simulink model "AutoFollow_Simulation"  (R2014a)
settings: Solver=ode45  StartTime=0.0  StopTime=50  FixedStep=0.05  MaxStep=0.06  RelTol=1e-3
model workspace (MAT data in the model file):
  Sig = Simulink.Signal
  Sig.DataType = 'auto'
  Sig.Dimensions = -1
  Sig.DimensionsMode = 'auto'
  Sig.Complexity = 'auto'
  Sig.SampleTime = -1
  Sig.SamplingMode = 'auto'
undefined symbols (not defined in the file or in its folder): IC, quadModel
libraries: simulink x4, commnoisgen2 x2
(part 1 of 2)
Description:
  | This is a configurable quadcopter simulation.
  | This Simulink model demonstates position control.
  | 
  | Additional quadcopter modeling and simulation materials available at:
  | github.com/dch33/Quad-Sim
  | 
  | Copyright (C) 2014 D. Hartman, K. Landis, S. Moreno, J. Kim, M. Mehrer
  | 
  | License:
  |     This program is free software: you can redistribute it and/or modify
  |     it under the terms of the GNU LESSER GENERAL PUBLIC LICENSE as published by
  |     the Free Software Foundation, either version 3 of the License, or
  |     (at your option) any later version.
  | 
  |     This program is distributed in the hope that it will be useful,
  |     but WITHOUT ANY WARRANTY; without even the implied warranty of
  |     MERCHANTABILITY or FITNESS FOR A PARTICULAR PURPOSE.  See the
  |     GNU General Public License for more details.
  | 
  |     You should have received a copy of the GNU LESSER GENERAL PUBLIC LICENSE
  |     along with this program.  If not, see <http://www.gnu.org/licenses/>.
settings Model: ModifiedComment=matthew -- Tue May 10 21:44:44 2016 -- Version 1.8  Creator=David Hartman  LastModifiedBy=jpacker
settings Model: ModifiedHistory=|
  | matthew -- Tue May 10 21:44:44 2016 -- Version 1.8
  | 
  | 
  | matthew -- Tue May 10 21:39:59 2016 -- Version 1.7
  | 
  | 
  | matthew -- Sun May 01 12:50:44 2016 -- Version 1.6
  | 
  | 
  | davidhartman -- Fri Jun 06 22:59:54 2014 -- Version 1.5
settings DataIOCC: LimitDataPoints=off  SignalLogging=off
settings OptimizationCC: InlineParams=on
settings DebuggingCC: MergeDetectMultiDrivingBlocksExec=error  UniqueDataStoreMsg=warning  StateNameClashWarn=warning  StrictBusMsg=ErrorOnBusTreatedAsVector

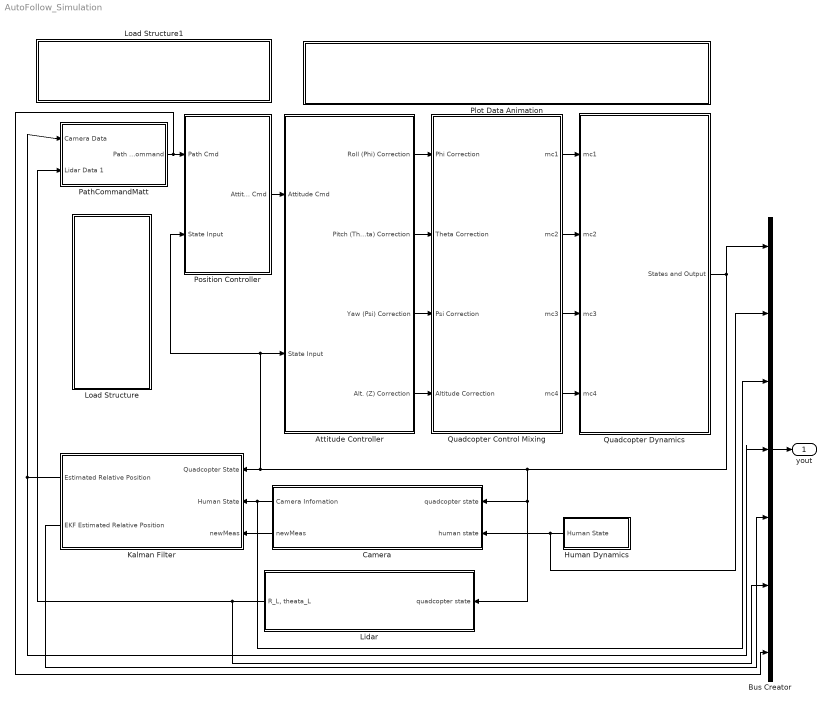
== system AutoFollow_Simulation ==
  Attitude Controller : Subsystem
  Bus Creator : BusCreator  Inputs=7
  Camera : Subsystem
  Human Dynamics : Subsystem
  Kalman Filter : Subsystem
  Lidar : Subsystem
  Load Structure : Subsystem
      settings: OpenFcn=|
      | uiopen('load')
      | if ((exist('IC')==1) && (exist('quadModel')==1) && (exist('path')==1))
      | set_param(bdroot, 'SimulationCommand', 'update')
      | end
      mask Display: fprintf('LOAD:\nTimeseries\nPath\nCommands,\nQuadcopter\nModel, Or\nInitial\nConditions');
  Load Structure1 : Subsystem
      settings: OpenFcn=|
      | if (exist('IC')==1 && exist('quadModel')==1 && exist('yout') && exist('tout'))
      | saveSimResults()
      | else
      | msgbox('No Data To Save!')
      | end
      mask Display: fprintf('SAVE:\nSimulation\nResults');
  "PathCommandMatt " : Subsystem
  Plot Data Animation : Subsystem
      settings: OpenFcn=|
      | if exist('QuadAnim4') == 2,
      |     if exist('yout')
      | 	run('QuadAnim4');
      |     else
      |     msgbox('Simulation must be run before data can be plotted.');
      |     end
      | else                                                                          msgbox('The desired GUI must be first added to MATLABs path.')
      | end
      mask Display: fprintf('OPEN GUI: Flight Animation')
  Position Controller : Subsystem
  Quadcopter Control Mixing : Subsystem
      mask Display:
      | modelLoaded = evalin('base','exist(''quadModel'',''var'')');
      | if (modelLoaded==1)
      |     if (evalin('base','quadModel.plusConfig'))
      |     fprintf([' \n' ' \n'  'Configuration "+"']);
      |     else if (~evalin('base','quadModel.plusConfig'))
      |         fprintf([' \n' ' \n' 'Configuration "X"']);
      |         end
      |     end
      | else
      |     fprintf([' \n' ' \n'  'Model Not Loaded']);
      | end
  Quadcopter Dynamics : Subsystem
  yout : Outport
  wires:
  Quadcopter Control Mixing/1(mc1) -> Quadcopter Dynamics/1(mc1)
  Quadcopter Control Mixing/2(mc2) -> Quadcopter Dynamics/2(mc2)
  Quadcopter Control Mixing/3(mc3) -> Quadcopter Dynamics/3(mc3)
  Quadcopter Control Mixing/4(mc4) -> Quadcopter Dynamics/4(mc4)
  Quadcopter Dynamics/1(States and Output) -> Lidar/1(quadcopter state), Camera/1(quadcopter state), Kalman Filter/1(Quadcopter State), Attitude Controller/2(State Input), Position Controller/2(State Input), Bus Creator/1
  Attitude Controller/1(Roll (Phi) Correction) -> Quadcopter Control Mixing/1(Phi Correction)
  Attitude Controller/2(Pitch (Theta) Correction) -> Quadcopter Control Mixing/2(Theta Correction)
  Attitude Controller/3(Yaw (Psi) Correction) -> Quadcopter Control Mixing/3(Psi Correction)
  Attitude Controller/4(Alt. (Z) Correction) -> Quadcopter Control Mixing/4(Altitude Correction)
  Position Controller/1(Attitude Cmd) -> Attitude Controller/1(Attitude Cmd)
  "PathCommandMatt "/1("Path Command ") -> Bus Creator/7, Position Controller/1(Path Cmd)
  Human Dynamics/1(Human State) -> Bus Creator/2, Camera/2(human state)
  Camera/1(Camera Infomation) -> Bus Creator/3, Kalman Filter/2(Human State)
  Bus Creator/1 -> yout/1
  Lidar/1("R_L, theata_L") -> "PathCommandMatt "/2(Lidar Data 1), Bus Creator/6
  Kalman Filter/1(Estimated Relative Position) -> "PathCommandMatt "/1("Camera Data "), Bus Creator/4
  Kalman Filter/2(EKF Estimated Relative Position) -> Bus Creator/5
  Camera/2(newMeas) -> Kalman Filter/3(newMeas)

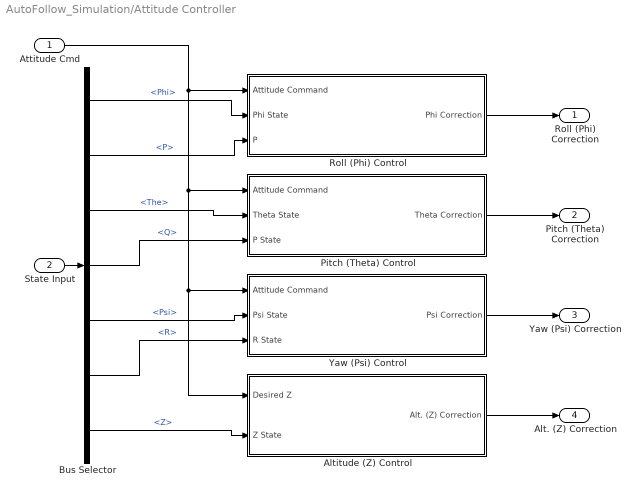
== system AutoFollow_Simulation/Attitude Controller ==
  Attitude Cmd : Inport
  State Input : Inport  Port=2
  Altitude (Z) Control : Subsystem  mask{Kpz=2, Kiz=1.1, Kdz=3.3, LimitOutput=on, USat=1, LSat=-1, GOffset=(sqrt((quadModel.mass*quadModel.g)/(4*quadModel.ct))-quadModel.b)/quadModel.cr}
      mask prompts: Kpz "Kp"; Kiz "Ki"; Kdz "Kd"; LimitOutput "Integral Saturation?"; USat "Upper saturation limit:"; LSat "Lower saturation limit:"; GOffset "Gravity Feedforward"
      mask help:
      | Adjust PID controller gains through this mask interface, or "look under mask" for more detailed adjustments.
      |
      | Note: Gravity Offset will not appear on block face as a value until simulation is run if it is the result of a formula involving the quadcopter model parameters.
      mask TypeOptions Kpz: Kpz/Gain
      mask TypeOptions Kiz: Kiz/Gain
      mask TypeOptions Kdz: Kdz/Gain
      mask TypeOptions LimitOutput:
      | Integrator
      | Limited/LimitOutput
      mask TypeOptions USat:
      | Integrator
      | Limited/UpperSaturationLimit
      mask TypeOptions LSat:
      | Integrator
      | Limited/LowerSaturationLimit
      mask TypeOptions GOffset: Gravity Offset (Level Flight)/Value
      mask Display:
      | fprintf(['Gravity Offset = ' num2str(GOffset) '\n' ...
      |     'Kp = ' num2str(Kpz) '\n' ...
      |     'Ki = ' num2str(Kiz) '\n' ...
      |     'Kd = ' num2str(Kdz) '\n' ...
      |     'Integral Saturation: ' LimitOutput]);
      | if strcmp(LimitOutput,'on')
      |     fprintf([' \n' ' \n' ' \n' ' \n' ' \n' '\n' ...
      |         'Limits: ' num2str(USat) ' to ' num2str(LSat)]);
      | end
  Bus Selector : BusSelector  OutputSignals=Phi,P,The,Q,Psi,R,Z
  Pitch (Theta) Control : Subsystem  mask{Kpt=2, Kit=1.1, Kdt=1.2, LimitOutput=on, USat=1, LSat=-1}
      mask prompts: Kpt "Kp"; Kit "Ki"; Kdt "Kd"; LimitOutput "Integral Saturation?"; USat "Upper saturation limit:"; LSat "Lower saturation limit:"
      mask help: Adjust PID controller gains through this mask interface, or "look under mask" for more detailed adjustments.
      mask TypeOptions Kpt: Kpt/Gain
      mask TypeOptions Kit: Kit/Gain
      mask TypeOptions Kdt: Kdt/Gain
      mask TypeOptions LimitOutput:
      | Integrator
      | Limited/LimitOutput
      mask TypeOptions USat:
      | Integrator
      | Limited/UpperSaturationLimit
      mask TypeOptions LSat:
      | Integrator
      | Limited/LowerSaturationLimit
      mask Display:
      | fprintf(['Kp = ' num2str(Kpt) '\n' ...
      |     'Ki = ' num2str(Kit) '\n' ...
      |     'Kd = ' num2str(Kdt) '\n' ...
      |     'Integral Saturation: ' LimitOutput]);
      | if strcmp(LimitOutput,'on')
      |     fprintf([' \n' ' \n' ' \n' ' \n' '\n' ...
      |         'Limits: ' num2str(USat) ' to ' num2str(LSat)]);
      | end
  "Roll (Phi) Control " : Subsystem  mask{Kpp=2.0, Kip=1.1, Kdp=1.2, LimitOutput=on, USat=1, LSat=-1}
      mask prompts: Kpp "Kp"; Kip "Ki"; Kdp "Kd"; LimitOutput "Integral Saturation:"; USat "Upper saturation limit:"; LSat "Lower saturation limit:"
      mask help:
      | Adjust PID controller gains through this mask interface, or "look under mask"
      | for more detailed adjustments.
      mask TypeOptions Kpp: Kpp/Gain
      mask TypeOptions Kip: Kip/Gain
      mask TypeOptions Kdp: Kdp/Gain
      mask TypeOptions LimitOutput:
      | Integrator
      | Limited/LimitOutput
      mask TypeOptions USat:
      | Integrator
      | Limited/UpperSaturationLimit
      mask TypeOptions LSat:
      | Integrator
      | Limited/LowerSaturationLimit
      mask Display:
      | fprintf(['Kp = ' num2str(Kpp) '\n' ...
      |     'Ki = ' num2str(Kip) '\n' ...
      |     'Kd = ' num2str(Kdp) '\n'...
      |     'Integral Saturation: ' LimitOutput]);
      | if strcmp(LimitOutput,'on')
      |     fprintf([' \n' ' \n' ' \n' ' \n' '\n' ...
      |         'Limits: ' num2str(USat) ' to ' num2str(LSat)]);
      | end
  Yaw (Psi) Control : Subsystem  mask{Kps=4, Kis=0.5, Kds=3.5, LimitOutput=on, USat=1, LSat=-1}
      mask prompts: Kps "Kp"; Kis "Ki"; Kds "Kd"; LimitOutput "Integral Saturation?"; USat "Upper saturation limit:"; LSat "Lower saturation limit:"
      mask help: Adjust PID controller gains through this mask interface, or "look under mask" for more detailed adjustments.
      mask TypeOptions Kps: Kps/Gain
      mask TypeOptions Kis: Kit/Gain
      mask TypeOptions Kds: Kds/Gain
      mask TypeOptions LimitOutput:
      | Integrator
      | Limited/LimitOutput
      mask TypeOptions USat:
      | Integrator
      | Limited/UpperSaturationLimit
      mask TypeOptions LSat:
      | Integrator
      | Limited/LowerSaturationLimit
      mask Display:
      | fprintf(['Kp = ' num2str(Kps) '\n' ...
      |     'Ki = ' num2str(Kis) '\n' ...
      |     'Kd = ' num2str(Kds) '\n' ...
      |     'Integral Saturation: ' LimitOutput]);
      | if strcmp(LimitOutput,'on')
      |     fprintf([' \n' ' \n' ' \n' ' \n' '\n' ...
      |         'Limits: ' num2str(USat) ' to ' num2str(LSat)]);
      | end
  Roll (Phi) Correction : Outport
  Pitch (Theta) Correction : Outport  Port=2
  Yaw (Psi) Correction : Outport  Port=3
  Alt. (Z) Correction : Outport  Port=4
  wires:
  "Roll (Phi) Control "/1(Phi Correction) -> Roll (Phi) Correction/1
  Bus Selector/1 -> "Roll (Phi) Control "/2(Phi State)  "<Phi>"
  State Input/1 -> Bus Selector/1
  Pitch (Theta) Control/1(Theta Correction) -> Pitch (Theta) Correction/1
  Yaw (Psi) Control/1(Psi Correction) -> Yaw (Psi) Correction/1
  Bus Selector/5 -> Yaw (Psi) Control/2(Psi State)  "<Psi>"
  Altitude (Z) Control/1(Alt. (Z) Correction) -> Alt. (Z) Correction/1
  Bus Selector/7 -> Altitude (Z) Control/2(Z State)  "<Z>"
  Attitude Cmd/1 -> Altitude (Z) Control/1(Desired Z), Yaw (Psi) Control/1(Attitude Command), Pitch (Theta) Control/1(Attitude Command), "Roll (Phi) Control "/1("Attitude Command ")
  Bus Selector/3 -> Pitch (Theta) Control/2(Theta State)  "<The>"
  Bus Selector/2 -> "Roll (Phi) Control "/3(P)  "<P>"
  Bus Selector/4 -> Pitch (Theta) Control/3(P State)  "<Q>"
  Bus Selector/6 -> Yaw (Psi) Control/3(R State)  "<R>"

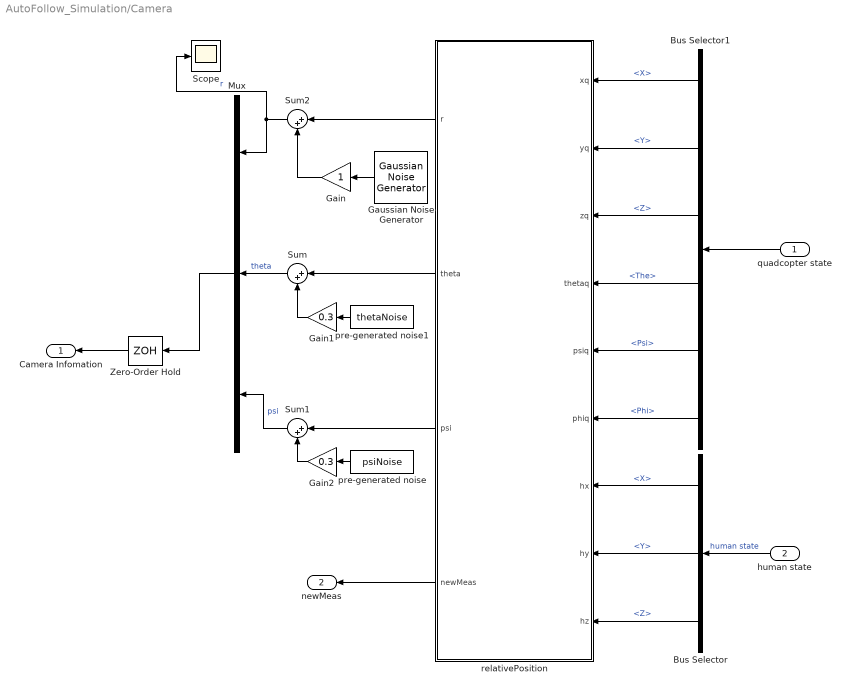
== system AutoFollow_Simulation/Camera ==
  quadcopter state : Inport
  human state : Inport  Port=2
  Bus Selector : BusSelector  OutputSignals=X,Y,Z
  Bus Selector1 : BusSelector  OutputSignals=X,Y,Z,The,Psi,Phi
  Gain : Gain
  Gain1 : Gain  Gain=0.3
  Gain2 : Gain  Gain=0.3
  Gaussian Noise Generator : commnoisgen2/Gaussian Noise Generator  m=0  d=1  s=35  Ts=1  frameBased=off  sampPerFrame=1  orient=off  outDataType=double
  Mux : Mux  Inputs=3
  Scope : Scope
  Sum : Sum  Inputs=|++
  Sum1 : Sum  Inputs=|++
  Sum2 : Sum  Inputs=|++
  Zero-Order Hold : ZeroOrderHold  SampleTime=0.05
  pre-generated noise : FromWorkspace  VariableName=psiNoise  Interpolate=off  OutputAfterFinalValue=Holding final value
  pre-generated noise1 : FromWorkspace  VariableName=thetaNoise  Interpolate=off  OutputAfterFinalValue=Holding final value
  relativePosition : MATLAB Function  TreatAsAtomicUnit=on
  Camera Infomation : Outport
  newMeas : Outport  Port=2
  wires:
  quadcopter state/1 -> Bus Selector1/1
  human state/1 -> Bus Selector/1  "human state"
  Bus Selector/3 -> relativePosition/9(hz)  "<Z>"
  Bus Selector1/1 -> relativePosition/1(xq)  "<X>"
  Bus Selector1/2 -> relativePosition/2(yq)  "<Y>"
  Bus Selector1/3 -> relativePosition/3(zq)  "<Z>"
  Bus Selector1/4 -> relativePosition/4(thetaq)  "<The>"
  Bus Selector1/5 -> relativePosition/5(psiq)  "<Psi>"
  Bus Selector1/6 -> relativePosition/6(phiq)  "<Phi>"
  Bus Selector/1 -> relativePosition/7(hx)  "<X>"
  Bus Selector/2 -> relativePosition/8(hy)  "<Y>"
  pre-generated noise1/1 -> Gain1/1
  pre-generated noise/1 -> Gain2/1
  relativePosition/1(r) -> Sum2/1
  relativePosition/2(theta) -> Sum/1
  relativePosition/3(psi) -> Sum1/1
  Gaussian Noise Generator/1 -> Gain/1
  Gain/1 -> Sum2/2
  Mux/1 -> Zero-Order Hold/1
  Sum2/1 -> Mux/1, Scope/1  "r"
  Sum/1 -> Mux/2  "theta"
  Sum1/1 -> Mux/3  "psi"
  Gain1/1 -> Sum/2
  Gain2/1 -> Sum1/2
  Zero-Order Hold/1 -> Camera Infomation/1
  relativePosition/4(newMeas) -> newMeas/1

== system AutoFollow_Simulation/Human Dynamics ==
  Path Command1 : Subsystem  mask{Interpolate=on, OutputAfterFinalValue=Holding final value}
      mask prompts: Interpolate "Interpolate X, Y, Z, and Psi command data?"; OutputAfterFinalValue "Form output after final data value by:"
      mask help:
      | Selecting the Interpolate data checkbox causes position commands to be
      | linearly interpolated. For additional options related to the Timeseries
      | "path" commands, look under the block and click on the Timeseries From
      | Workspace blocks.
      mask TypeOptions Interpolate: X Timeseries From Wkspace/Interpolate | Y Timeseries From Wkspace/Interpolate | Z Timeseries From Wkspace/Interpolate | Psi Timeseries From Wkspace/Interpolate
      mask TypeOptions OutputAfterFinalValue: X Timeseries From Wkspace/OutputAfterFinalValue | Y Timeseries From Wkspace/OutputAfterFinalValue | Z Timeseries From Wkspace/OutputAfterFinalValue | Psi Timeseries From Wkspace/OutputAfterFinalValue
  Human State : Outport
  wires:
  Path Command1/1("Path Command ") -> Human State/1

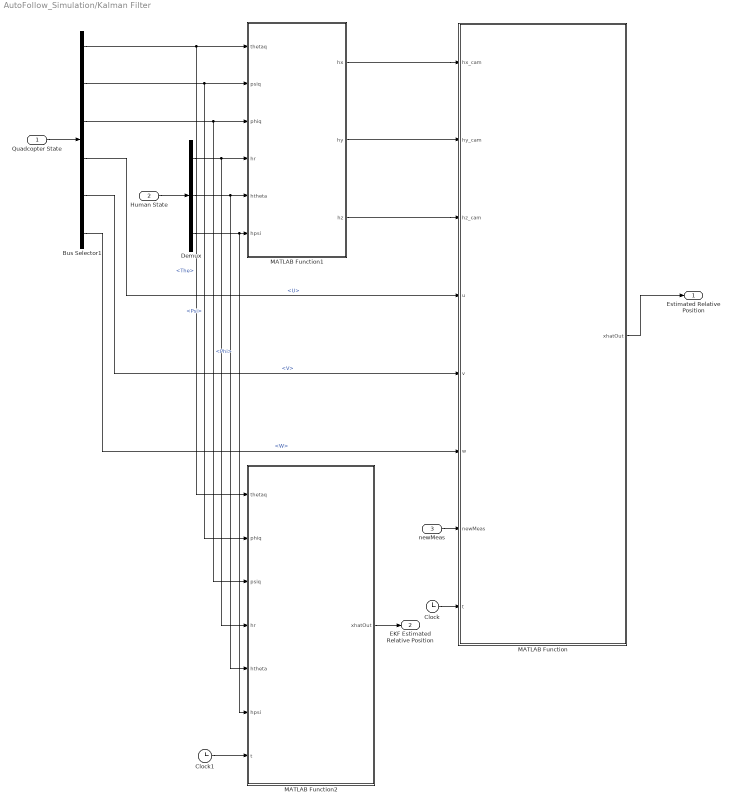
== system AutoFollow_Simulation/Kalman Filter ==
  Quadcopter State : Inport
  Human State : Inport  Port=2
  newMeas : Inport  Port=3
  Bus Selector1 : BusSelector  OutputSignals=The,Psi,Phi,U,V,W
  Clock : Clock
  Clock1 : Clock
  Demux : Demux  Outputs=3
  MATLAB Function : MATLAB Function  TreatAsAtomicUnit=on
  MATLAB Function1 : MATLAB Function  TreatAsAtomicUnit=on
  MATLAB Function2 : MATLAB Function  TreatAsAtomicUnit=on
  Estimated Relative Position : Outport
  EKF Estimated Relative Position : Outport  Port=2
  wires:
  Quadcopter State/1 -> Bus Selector1/1
  Human State/1 -> Demux/1
  Bus Selector1/2 -> MATLAB Function1/2(psiq), MATLAB Function2/2(phiq)  "<Psi>"
  Bus Selector1/1 -> MATLAB Function1/1(thetaq), MATLAB Function2/1(thetaq)  "<The>"
  Bus Selector1/3 -> MATLAB Function2/3(psiq), MATLAB Function1/3(phiq)  "<Phi>"
  Demux/1 -> MATLAB Function2/4(hr), MATLAB Function1/4(hr)
  Demux/2 -> MATLAB Function2/5(htheta), MATLAB Function1/5(htheta)
  Demux/3 -> MATLAB Function2/6(hpsi), MATLAB Function1/6(hpsi)
  MATLAB Function1/3(hz) -> MATLAB Function/3(hz_cam)
  MATLAB Function1/2(hy) -> MATLAB Function/2(hy_cam)
  MATLAB Function1/1(hx) -> MATLAB Function/1(hx_cam)
  Clock/1 -> MATLAB Function/8(t)
  MATLAB Function/1(xhatOut) -> Estimated Relative Position/1
  Clock1/1 -> MATLAB Function2/7(t)
  MATLAB Function2/1(xhatOut) -> EKF Estimated Relative Position/1
  Bus Selector1/4 -> MATLAB Function/4(u)  "<U>"
  Bus Selector1/5 -> MATLAB Function/5(v)  "<V>"
  Bus Selector1/6 -> MATLAB Function/6(w)  "<W>"
  newMeas/1 -> MATLAB Function/7(newMeas)

== system AutoFollow_Simulation/Lidar ==
  quadcopter state : Inport
  Bus Selector1 : BusSelector  OutputSignals=X,Y
  Clock : Clock
  Gain : Gain  Commented=on  Gain=3
  Gaussian Noise Generator : commnoisgen2/Gaussian Noise Generator  Commented=on  m=0  d=1  s=35  Ts=1  frameBased=off  sampPerFrame=1  orient=off  outDataType=double
  MATLAB Function : MATLAB Function  TreatAsAtomicUnit=on
  Mux : Mux  Inputs=2
  pre-generated noise1 : FromWorkspace  Commented=on  VariableName=thetaNoise  Interpolate=off  OutputAfterFinalValue=Holding final value
  "R_L, theata_L" : Outport
  wires:
  quadcopter state/1 -> Bus Selector1/1
  Bus Selector1/1 -> MATLAB Function/1(xq)  "<X>"
  Bus Selector1/2 -> MATLAB Function/2(yq)  "<Y>"
  pre-generated noise1/1 -> ?
  MATLAB Function/1(r) -> Mux/1
  MATLAB Function/2(theta) -> Mux/2
  Gaussian Noise Generator/1 -> Gain/1
  Gain/1 -> ?
  Mux/1 -> "R_L, theata_L"/1
  Clock/1 -> MATLAB Function/3(t)

== system AutoFollow_Simulation/Load Structure ==

== system AutoFollow_Simulation/Load Structure1 ==

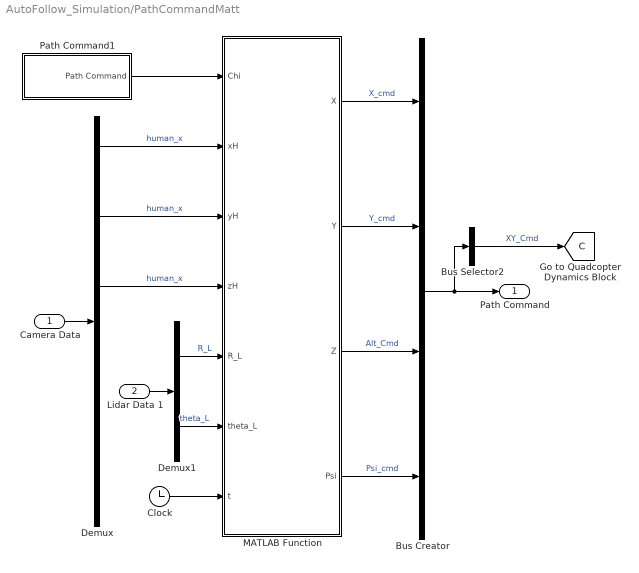
== system AutoFollow_Simulation/PathCommandMatt  ==
  "Camera Data " : Inport
  Lidar Data 1 : Inport  Port=2
  Bus Creator : BusCreator
  Bus Selector2 : BusSelector  OutputSignals=X_cmd,Y_cmd  OutputAsBus=on
  Clock : Clock
  Demux : Demux  Outputs=6
  Demux1 : Demux  Outputs=2
  MATLAB Function : MATLAB Function  TreatAsAtomicUnit=on
  Path Command1 : Subsystem  mask{Interpolate=on, OutputAfterFinalValue=Holding final value}
      mask prompts: Interpolate "Interpolate X, Y, Z, and Psi command data?"; OutputAfterFinalValue "Form output after final data value by:"
      mask help:
      | Selecting the Interpolate data checkbox causes position commands to be
      | linearly interpolated. For additional options related to the Timeseries
      | "path" commands, look under the block and click on the Timeseries From
      | Workspace blocks.
      mask TypeOptions Interpolate: X Timeseries From Wkspace/Interpolate | Y Timeseries From Wkspace/Interpolate | Z Timeseries From Wkspace/Interpolate | Psi Timeseries From Wkspace/Interpolate
      mask TypeOptions OutputAfterFinalValue: X Timeseries From Wkspace/OutputAfterFinalValue | Y Timeseries From Wkspace/OutputAfterFinalValue | Z Timeseries From Wkspace/OutputAfterFinalValue | Psi Timeseries From Wkspace/OutputAfterFinalValue
  "Path Command " : Outport
  tag scope: C=global
  wires:
  Bus Selector2/1 -> [C]  "XY_Cmd"
  MATLAB Function/1(X) -> Bus Creator/1  "X_cmd"
  MATLAB Function/2(Y) -> Bus Creator/2  "Y_cmd"
  MATLAB Function/3(Z) -> Bus Creator/3  "Alt_Cmd"
  MATLAB Function/4(Psi) -> Bus Creator/4  "Psi_cmd"
  Bus Creator/1 -> "Path Command "/1, Bus Selector2/1
  "Camera Data "/1 -> Demux/1
  Demux/1 -> MATLAB Function/2(xH)  "human_x"
  Demux/3 -> MATLAB Function/4(zH)  "human_x"
  Demux/2 -> MATLAB Function/3(yH)  "human_x"
  Clock/1 -> MATLAB Function/7(t)
  Path Command1/1("Path Command ") -> MATLAB Function/1(Chi)
  Lidar Data 1/1 -> Demux1/1
  Demux1/1 -> MATLAB Function/5(R_L)  "R_L"
  Demux1/2 -> MATLAB Function/6(theta_L)  "theta_L"

== system AutoFollow_Simulation/Plot Data Animation ==

== system AutoFollow_Simulation/Position Controller ==
  note: made a change
  note: Inertial-frame velocity is used as the state to be controlled,
      | (as this is what is controlled by attitude)
      | thus we find position error in the body frame
      | and map this to a body frame desired velocity. This desired
      | velocity is then mapped to a desired attitude.
  Path Cmd : Inport
  State Input : Inport  Port=2
  Bus Creator : BusCreator
  Bus Selector : BusSelector  OutputSignals=X_cmd,Y_cmd,Alt_Cmd,Psi_cmd
  Bus Selector1 : BusSelector  OutputSignals=X,Y,Psi,U,V
  Error Rotations : Subsystem
  Phi Command Control : Subsystem  mask{Kp=0.32, Kd=0.1, ASat=12*pi/180}
      mask prompts: Kp "Proportional Gain"; Kd "Derivative Gain"; ASat "Attitude Limit (+/- radians):"
      mask TypeOptions Kp: Kpp/Gain
      mask TypeOptions Kd: Kdp/Gain
      mask TypeOptions ASat: Attitude Limits_Phi/UpperLimit
      mask Display:
      | fprintf(['Kp = ' num2str(Kp) '\n' ...
      |     'Kd = ' num2str(Kd) '\n' ...
      |     'Attitude Limit (+/-): ' num2str(ASat*180/pi) '°']);
  Theta Command Control : Subsystem  mask{Kp=0.32, Kd=0.10, ASat=12*pi/180}
      mask prompts: Kp "Proportional Gain:"; Kd "Derivative Gain"; ASat "Attitude Limit (+/- radians):"
      mask TypeOptions Kp: Kpt/Gain
      mask TypeOptions Kd: Kdt/Gain
      mask TypeOptions ASat: Attitude Limits_Theta/UpperLimit
      mask Display:
      | fprintf(['Kp = ' num2str(Kp) '\n' ...
      |     'Kd = ' num2str(Kd) '\n' ...
      |     'Attitude Limit (+/-): ' num2str(ASat*180/pi) '°']);
  Attitude Cmd : Outport
  tag scope: A=global
  wires:
  Bus Selector1/5 -> Phi Command Control/2(Yb Velocity)  "<V>"
  State Input/1 -> Bus Selector1/1
  Path Cmd/1 -> Bus Selector/1
  Bus Creator/1 -> Attitude Cmd/1, [A]  "Attitude_Cmd"
  Bus Selector1/1 -> Error Rotations/3(X)  "<X>"
  Bus Selector1/2 -> Error Rotations/4(Y)  "<Y>"
  Bus Selector1/3 -> Error Rotations/5(Psi)  "<Psi>"
  Error Rotations/1(X Error in body Frame) -> Theta Command Control/1(Desired Xb Velocity)  "Desired velocity in Xb"
  Bus Selector1/4 -> Theta Command Control/2(Xb Velocity)  "<U>"
  Theta Command Control/1(The_cmd) -> Bus Creator/2  "The_cmd"
  Error Rotations/2(Y Error in Body Frame) -> Phi Command Control/1(Desired Yb Velocity)  "Desired Velocity in Yb"
  Phi Command Control/1(Phi_cmd) -> Bus Creator/1  "Phi_cmd"
  Bus Selector/4 -> Bus Creator/3  "<Psi_cmd>"
  Bus Selector/3 -> Bus Creator/4  "<Alt_Cmd>"
  Bus Selector/2 -> Error Rotations/2(Y_cmd)  "<Y_cmd>"
  Bus Selector/1 -> Error Rotations/1(X_cmd)  "<X_cmd>"

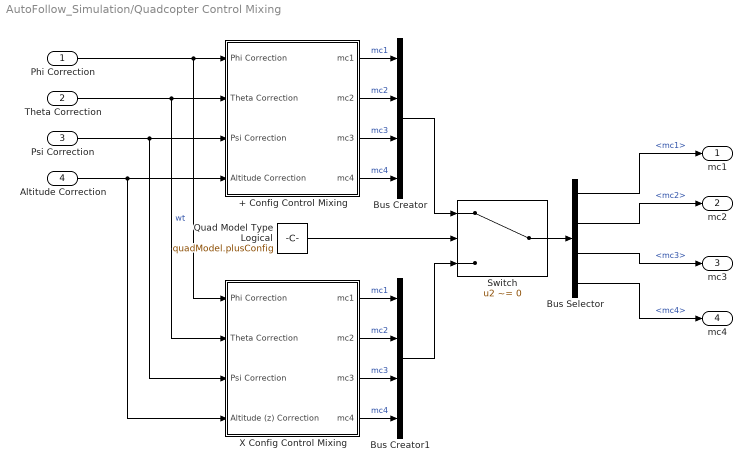
== system AutoFollow_Simulation/Quadcopter Control Mixing ==
  Phi Correction : Inport
  Theta Correction : Inport  Port=2
  Psi Correction : Inport  Port=3
  Altitude Correction : Inport  Port=4
  + Config Control Mixing : Subsystem
  Bus Creator : BusCreator
  Bus Creator1 : BusCreator
  Bus Selector : BusSelector  OutputSignals=mc1,mc2,mc3,mc4
  Quad Model Type Logical : Constant  Value=quadModel.plusConfig
  Switch : Switch  Criteria=u2 ~= 0
  X Config Control Mixing : Subsystem
  mc1 : Outport
  mc2 : Outport  Port=2
  mc3 : Outport  Port=3
  mc4 : Outport  Port=4
  wires:
  Phi Correction/1 -> X Config Control Mixing/1(Phi Correction), + Config Control Mixing/1(Phi Correction)
  Theta Correction/1 -> X Config Control Mixing/2(Theta Correction), + Config Control Mixing/2(Theta Correction)  "wt"
  Psi Correction/1 -> X Config Control Mixing/3(Psi Correction), + Config Control Mixing/3(Psi Correction)
  Altitude Correction/1 -> X Config Control Mixing/4(Altitude (z) Correction), + Config Control Mixing/4(Altitude Correction)
  + Config Control Mixing/1(mc1) -> Bus Creator/1  "mc1"
  + Config Control Mixing/2(mc2) -> Bus Creator/2  "mc2"
  + Config Control Mixing/3(mc3) -> Bus Creator/3  "mc3"
  + Config Control Mixing/4(mc4) -> Bus Creator/4  "mc4"
  Bus Creator/1 -> Switch/1
  X Config Control Mixing/1(mc1) -> Bus Creator1/1  "mc1"
  X Config Control Mixing/2(mc2) -> Bus Creator1/2  "mc2"
  X Config Control Mixing/3(mc3) -> Bus Creator1/3  "mc3"
  X Config Control Mixing/4(mc4) -> Bus Creator1/4  "mc4"
  Bus Creator1/1 -> Switch/3
  Bus Selector/1 -> mc1/1  "<mc1>"
  Bus Selector/2 -> mc2/1  "<mc2>"
  Bus Selector/3 -> mc3/1  "<mc3>"
  Bus Selector/4 -> mc4/1  "<mc4>"
  Quad Model Type Logical/1 -> Switch/2
  Switch/1 -> Bus Selector/1

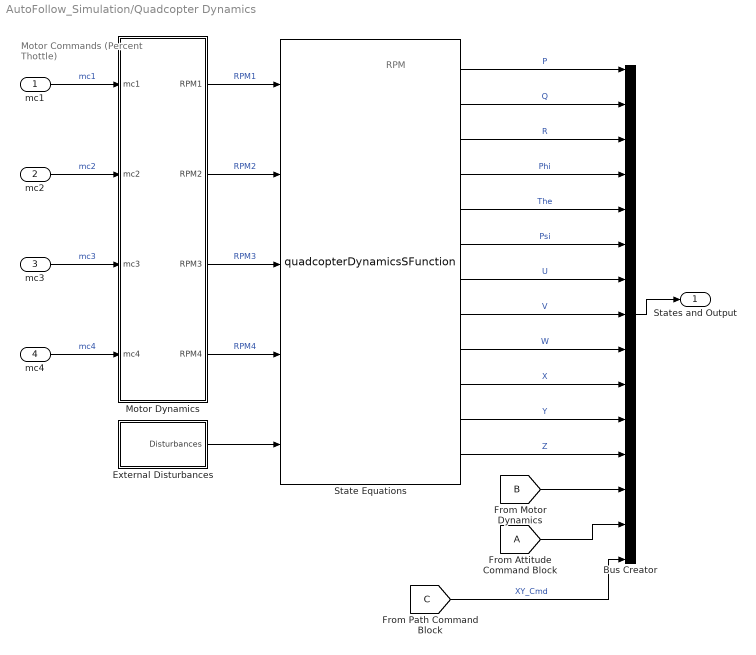
== system AutoFollow_Simulation/Quadcopter Dynamics ==
  note: RPM
  note: Motor Commands
      | (Percent Thottle)
  mc1 : Inport
  mc2 : Inport  Port=2
  mc3 : Inport  Port=3
  mc4 : Inport  Port=4
  Bus Creator : BusCreator  Inputs='P','Q','R','Phi','The','Psi','U','V','W','X','Y','Z','mc and RPM','Attitude_Cmd','XY_Cmd'
  External Disturbances : Subsystem
  Motor Dynamics : Subsystem
  State Equations : M-S-Function  FunctionName=quadcopterDynamicsSFunction  Parameters=quadModel, IC
      mask Display:
      | port_label('input', 1, 'RPM1')
      | port_label('input', 2, 'RPM2')
      | port_label('input', 3, 'RPM3')
      | port_label('input', 4, 'RPM4')
      | port_label('input', 5, 'Disturbances')
      | port_label('output', 1, 'P')
      | port_label('output', 2, 'Q')
      | port_label('output', 3, 'R')
      | port_label('output', 4, 'Phi')
      | port_label('output', 5, 'The')
      | port_label('output', 6, 'Psi')
      | port_label('output', 7, 'U')
      | port_label('output', 8, 'V')
      | port_label('output', 9, 'W')
      | port_label('output', 10, 'X')
      | port_label('output', 11, 'Y')
      | port_label('output', 12, 'Z')
  States and Output : Outport
  wires:
  State Equations/1 -> Bus Creator/1  "P"
  State Equations/2 -> Bus Creator/2  "Q"
  State Equations/3 -> Bus Creator/3  "R"
  State Equations/4 -> Bus Creator/4  "Phi"
  State Equations/5 -> Bus Creator/5  "The"
  State Equations/6 -> Bus Creator/6  "Psi"
  State Equations/7 -> Bus Creator/7  "U"
  State Equations/8 -> Bus Creator/8  "V"
  State Equations/9 -> Bus Creator/9  "W"
  State Equations/10 -> Bus Creator/10  "X"
  State Equations/11 -> Bus Creator/11  "Y"
  State Equations/12 -> Bus Creator/12  "Z"
  Bus Creator/1 -> States and Output/1
  Motor Dynamics/1(RPM1) -> State Equations/1  "RPM1"
  Motor Dynamics/2(RPM2) -> State Equations/2  "RPM2"
  Motor Dynamics/3(RPM3) -> State Equations/3  "RPM3"
  Motor Dynamics/4(RPM4) -> State Equations/4  "RPM4"
  mc1/1 -> Motor Dynamics/1(mc1)  "mc1"
  mc4/1 -> Motor Dynamics/4(mc4)  "mc4"
  mc3/1 -> Motor Dynamics/3(mc3)  "mc3"
  mc2/1 -> Motor Dynamics/2(mc2)  "mc2"
  External Disturbances/1("Disturbances ") -> State Equations/5
  [A] -> Bus Creator/14
  [B] -> Bus Creator/13
  [C] -> Bus Creator/15  "XY_Cmd"

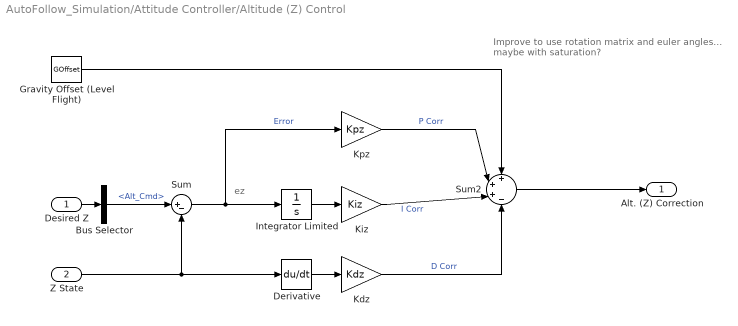
== system AutoFollow_Simulation/Attitude Controller/Altitude (Z) Control ==
  note: Improve to use rotation matrix and euler angles...
      | maybe with saturation?
  note: ez
  Desired Z : Inport
  Z State : Inport  Port=2
  Bus Selector : BusSelector  OutputSignals=Alt_Cmd
  Derivative : Derivative
  Gravity Offset (Level Flight) : Constant  Value=GOffset
  Integrator Limited : Integrator  LimitOutput=on  UpperSaturationLimit=USat  LowerSaturationLimit=LSat
  Kdz : Gain  Gain=Kdz
  Kiz : Gain  Gain=Kiz
  Kpz : Gain  Gain=Kpz
  Sum : Sum  Inputs=|+-
  Sum2 : Sum  Inputs=+++-
  Alt. (Z) Correction : Outport
  wires:
  Gravity Offset (Level Flight)/1 -> Sum2/1
  Desired Z/1 -> Bus Selector/1
  Z State/1 -> Derivative/1, Sum/2
  Sum2/1 -> Alt. (Z) Correction/1
  Kpz/1 -> Sum2/2  "P Corr"
  Sum/1 -> Integrator Limited/1, Kpz/1  "Error"
  Kiz/1 -> Sum2/3  "I Corr"
  Kdz/1 -> Sum2/4  "D Corr"
  Integrator Limited/1 -> Kiz/1
  Bus Selector/1 -> Sum/1  "<Alt_Cmd>"
  Derivative/1 -> Kdz/1

== system AutoFollow_Simulation/Attitude Controller/Pitch (Theta) Control ==
  Attitude Command : Inport
  Theta State : Inport  Port=2
  P State : Inport  Port=3
  Bus Selector : BusSelector  OutputSignals=The_cmd
  Integrator Limited : Integrator  LimitOutput=on  UpperSaturationLimit=USat  LowerSaturationLimit=LSat
  Kdt : Gain  Gain=Kdt
  Kit : Gain  Gain=Kit
  Kpt : Gain  Gain=Kpt
  Sum : Sum  Inputs=|+-
  Sum1 : Sum  Inputs=++-
  Theta Correction : Outport
  wires:
  Sum/1 -> Integrator Limited/1, Kpt/1  "Error"
  Attitude Command/1 -> Bus Selector/1
  Theta State/1 -> Sum/2
  Sum1/1 -> Theta Correction/1
  Kpt/1 -> Sum1/1  "P Corr"
  Kdt/1 -> Sum1/3  "D Corr"
  Kit/1 -> Sum1/2  "I Corr"
  Integrator Limited/1 -> Kit/1
  Bus Selector/1 -> Sum/1  "<The_cmd>"
  P State/1 -> Kdt/1

== system AutoFollow_Simulation/Attitude Controller/Roll (Phi) Control  ==
  "Attitude Command " : Inport
  Phi State : Inport  Port=2
  P : Inport  Port=3
  Bus Selector : BusSelector  OutputSignals=Phi_cmd
  Integrator Limited : Integrator  LimitOutput=on  UpperSaturationLimit=USat  LowerSaturationLimit=LSat
  Kdp : Gain  Gain=Kdp
  Kip : Gain  Gain=Kip
  Kpp : Gain  Gain=Kpp
  Sum : Sum  Inputs=|+-
  Sum1 : Sum  Inputs=++-
  Phi Correction : Outport
  wires:
  Sum/1 -> Integrator Limited/1, Kpp/1  "Error"
  Phi State/1 -> Sum/2
  Sum1/1 -> Phi Correction/1
  Kpp/1 -> Sum1/1  "P Corr"
  Kdp/1 -> Sum1/3  "D Corr"
  Kip/1 -> Sum1/2  "I Corr"
  Integrator Limited/1 -> Kip/1
  "Attitude Command "/1 -> Bus Selector/1
  Bus Selector/1 -> Sum/1  "<Phi_cmd>"
  P/1 -> Kdp/1

== system AutoFollow_Simulation/Attitude Controller/Yaw (Psi) Control ==
  Attitude Command : Inport
  Psi State : Inport  Port=2
  R State : Inport  Port=3
  Bus Selector : BusSelector  OutputSignals=Psi_cmd
  Integrator Limited : Integrator  LimitOutput=on  UpperSaturationLimit=USat  LowerSaturationLimit=LSat
  Kds : Gain  Gain=Kds
  Kit : Gain  Gain=Kis
  Kps : Gain  Gain=Kps
  Sum : Sum  Inputs=|+-
  Sum1 : Sum  Inputs=++-
  Psi Correction : Outport
  wires:
  Sum/1 -> Integrator Limited/1, Kps/1  "Error"
  Attitude Command/1 -> Bus Selector/1
  Sum1/1 -> Psi Correction/1
  Psi State/1 -> Sum/2
  Kps/1 -> Sum1/1  "P Corr"
  Kds/1 -> Sum1/3  "D Corr"
  Kit/1 -> Sum1/2  "I Corr"
  Integrator Limited/1 -> Kit/1
  Bus Selector/1 -> Sum/1  "<Psi_cmd>"
  R State/1 -> Kds/1

== system AutoFollow_Simulation/Human Dynamics/Path Command1 ==
  Bus Creator : BusCreator
  Psi Timeseries From Wkspace : FromWorkspace  VariableName=human.psi  SampleTime=0  OutputAfterFinalValue=Holding final value
  X Timeseries From Wkspace : FromWorkspace  VariableName=human.x  SampleTime=0  OutputAfterFinalValue=Holding final value
  Y Timeseries From Wkspace : FromWorkspace  VariableName=human.y  SampleTime=0  OutputAfterFinalValue=Holding final value
  Z Timeseries From Wkspace : FromWorkspace  VariableName=human.z  SampleTime=0  OutputAfterFinalValue=Holding final value
  "Path Command " : Outport
  wires:
  X Timeseries From Wkspace/1 -> Bus Creator/1  "X"
  Y Timeseries From Wkspace/1 -> Bus Creator/2  "Y"
  Z Timeseries From Wkspace/1 -> Bus Creator/3  "Z"
  Psi Timeseries From Wkspace/1 -> Bus Creator/4  "Psi"
  Bus Creator/1 -> "Path Command "/1

== system AutoFollow_Simulation/PathCommandMatt /Path Command1 ==
  X Timeseries From Wkspace : FromWorkspace  VariableName=Chi  SampleTime=0  OutputAfterFinalValue=Holding final value
  "Path Command " : Outport
  wires:
  X Timeseries From Wkspace/1 -> "Path Command "/1  "Chi cmd"

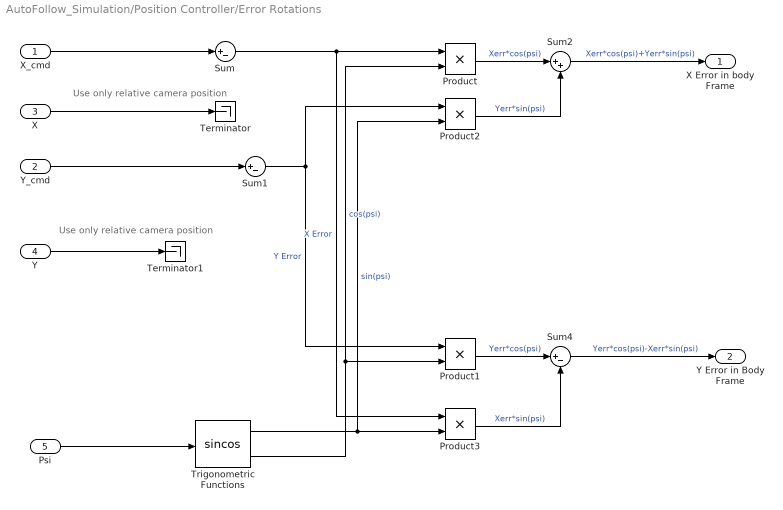
== system AutoFollow_Simulation/Position Controller/Error Rotations ==
  note: Use only relative camera position
  note: Use only relative camera position
  X_cmd : Inport
  Y_cmd : Inport  Port=2
  X : Inport  Port=3
  Y : Inport  Port=4
  Psi : Inport  Port=5
  Product{,1..3} (4 alike) : Product
  Sum : Sum  Inputs=|+-
  Sum1 : Sum  Inputs=|+-
  Sum2 : Sum  Inputs=|++
  Sum4 : Sum  Inputs=|+-
  Terminator : Terminator
  Terminator1 : Terminator
  Trigonometric Functions : Trigonometry  Operator=sincos
  X Error in body Frame : Outport
  Y Error in Body Frame : Outport  Port=2
  wires:
  Sum4/1 -> Y Error in Body Frame/1  "Yerr*cos(psi)-Xerr*sin(psi)"
  Product3/1 -> Sum4/2  "Xerr*sin(psi)"
  Sum1/1 -> Product2/1, Product1/1  "Y Error"
  Trigonometric Functions/1 -> Product2/2, Product3/2  "sin(psi)"
  Sum2/1 -> X Error in body Frame/1  "Xerr*cos(psi)+Yerr*sin(psi)"
  Y_cmd/1 -> Sum1/1
  X_cmd/1 -> Sum/1
  X/1 -> Terminator/1
  Y/1 -> Terminator1/1
  Sum/1 -> Product3/1, Product/1  "X Error"
  Trigonometric Functions/2 -> Product/2, Product1/2  "cos(psi)"
  Product/1 -> Sum2/1  "Xerr*cos(psi)"
  Product2/1 -> Sum2/2  "Yerr*sin(psi)"
  Product1/1 -> Sum4/1  "Yerr*cos(psi)"
  Psi/1 -> Trigonometric Functions/1

== system AutoFollow_Simulation/Position Controller/Phi Command Control ==
  note: -1 Gain is required because a "negative"
      | angle of Phi induces a positive velocity
      | in the body frame y direction!
  Desired Yb Velocity : Inport
  Yb Velocity : Inport  Port=2
  Attitude Limits_Phi : Saturate  UpperLimit=ASat  LowerLimit=-ASat
  Gain : Gain  Gain=-1
  Kdp : Gain  Gain=Kd
  Kpp : Gain  Gain=Kp
  Sum3 : Sum  Inputs=|+-
  Sum6 : Sum  Inputs=|+-
  V Derivative : Derivative
  Phi_cmd : Outport
  wires:
  V Derivative/1 -> Kdp/1
  Attitude Limits_Phi/1 -> Phi_cmd/1  "Phi_cmd"
  Sum6/1 -> Gain/1
  Kpp/1 -> Sum6/1
  Sum3/1 -> Kpp/1  "Velocity Error"
  Yb Velocity/1 -> V Derivative/1, Sum3/2
  Desired Yb Velocity/1 -> Sum3/1
  Gain/1 -> Attitude Limits_Phi/1
  Kdp/1 -> Sum6/2

== system AutoFollow_Simulation/Position Controller/Theta Command Control ==
  Desired Xb Velocity : Inport
  Xb Velocity : Inport  Port=2
  Attitude Limits_Theta : Saturate  UpperLimit=ASat  LowerLimit=-ASat
  Kdt : Gain  Gain=Kd
  Kpt : Gain  Gain=Kp
  Sum3 : Sum  Inputs=|+-
  Sum6 : Sum  Inputs=|+-
  U Derivative : Derivative
  The_cmd : Outport
  wires:
  Kdt/1 -> Sum6/2
  U Derivative/1 -> Kdt/1
  Attitude Limits_Theta/1 -> The_cmd/1  "The_cmd"
  Sum6/1 -> Attitude Limits_Theta/1
  Kpt/1 -> Sum6/1
  Sum3/1 -> Kpt/1  "Velocity Error"
  Xb Velocity/1 -> U Derivative/1, Sum3/2
  Desired Xb Velocity/1 -> Sum3/1

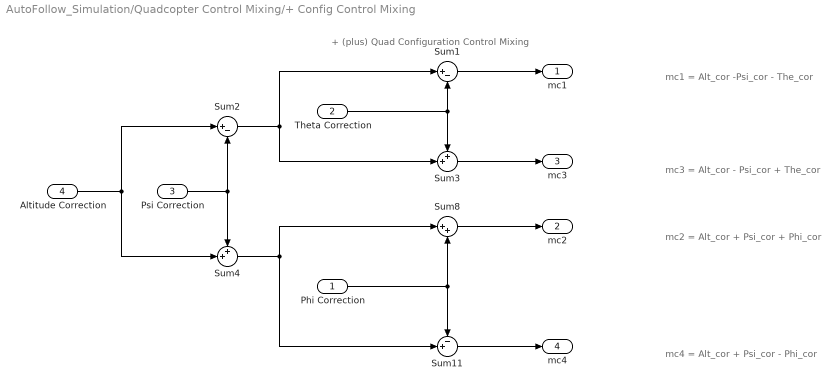
== system AutoFollow_Simulation/Quadcopter Control Mixing/+ Config Control Mixing ==
  note: mc2 = Alt_cor + Psi_cor + Phi_cor
  note: + (plus) Quad Configuration Control Mixing
  note: mc4 = Alt_cor + Psi_cor - Phi_cor
  note: mc3 = Alt_cor - Psi_cor + The_cor
  note: mc1 = Alt_cor -Psi_cor - The_cor
  Phi Correction : Inport
  Theta Correction : Inport  Port=2
  Psi Correction : Inport  Port=3
  Altitude Correction : Inport  Port=4
  Sum1 : Sum  Inputs=|+-
  Sum11 : Sum  Inputs=-+|
  Sum2 : Sum  Inputs=|+-
  Sum3 : Sum  Inputs=++|
  Sum4 : Sum  Inputs=++|
  Sum8 : Sum  Inputs=|++
  mc1 : Outport
  mc2 : Outport  Port=2
  mc3 : Outport  Port=3
  mc4 : Outport  Port=4
  wires:
  Theta Correction/1 -> Sum1/2, Sum3/1
  Altitude Correction/1 -> Sum2/1, Sum4/2
  Sum2/1 -> Sum3/2, Sum1/1
  Psi Correction/1 -> Sum4/1, Sum2/2
  Sum4/1 -> Sum11/2, Sum8/1
  Phi Correction/1 -> Sum8/2, Sum11/1
  Sum1/1 -> mc1/1
  Sum3/1 -> mc3/1
  Sum8/1 -> mc2/1
  Sum11/1 -> mc4/1

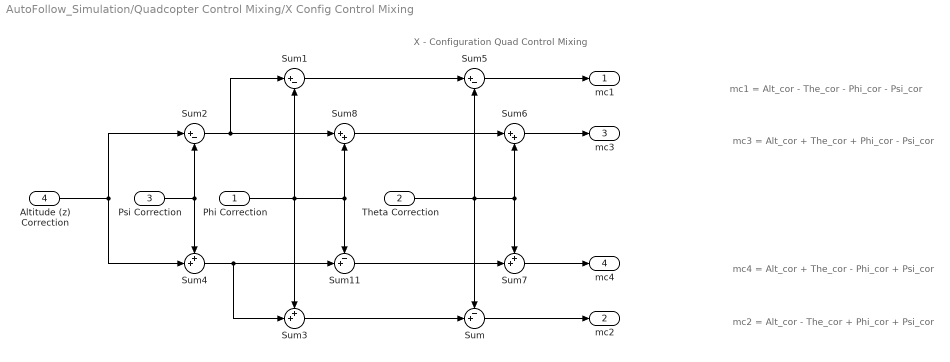
== system AutoFollow_Simulation/Quadcopter Control Mixing/X Config Control Mixing ==
  note: mc1 = Alt_cor - The_cor - Phi_cor - Psi_cor
  note: X - Configuration Quad Control Mixing
  note: mc3 = Alt_cor + The_cor + Phi_cor - Psi_cor
  note: mc2 = Alt_cor - The_cor + Phi_cor + Psi_cor
  note: mc4 = Alt_cor + The_cor - Phi_cor + Psi_cor
  Phi Correction : Inport
  Theta Correction : Inport  Port=2
  Psi Correction : Inport  Port=3
  Altitude (z) Correction : Inport  Port=4
  Sum : Sum  Inputs=-+|
  Sum1 : Sum  Inputs=|+-
  Sum11 : Sum  Inputs=-+|
  Sum2 : Sum  Inputs=|+-
  Sum3 : Sum  Inputs=++|
  Sum4 : Sum  Inputs=++|
  Sum5 : Sum  Inputs=|+-
  Sum6 : Sum  Inputs=|++
  Sum7 : Sum  Inputs=++|
  Sum8 : Sum  Inputs=|++
  mc1 : Outport
  mc2 : Outport  Port=2
  mc3 : Outport  Port=3
  mc4 : Outport  Port=4
  wires:
  Sum2/1 -> Sum8/1, Sum1/1
  Psi Correction/1 -> Sum4/1, Sum2/2
  Phi Correction/1 -> Sum3/1, Sum1/2, Sum8/2, Sum11/1
  Sum4/1 -> Sum3/2, Sum11/2
  Sum3/1 -> Sum/2
  Theta Correction/1 -> Sum7/1, Sum6/2, Sum5/2, Sum/1
  Sum1/1 -> Sum5/1
  Sum8/1 -> Sum6/1
  Sum11/1 -> Sum7/2
  Sum5/1 -> mc1/1
  Sum6/1 -> mc3/1
  Sum7/1 -> mc4/1
  Altitude (z) Correction/1 -> Sum2/1, Sum4/2
  Sum/1 -> mc2/1

== system AutoFollow_Simulation/Quadcopter Dynamics/External Disturbances ==
  note: Note: Torques are in units of N*m, Forces in N
      | Torques are applied to the BODY coordinate system.
      | Forces are applied from the WORLD coordinate system!
      | This can be changed by adjusting the equations within the S-function.
  Bus Creator : BusCreator  Inputs=6
  Bus to Vector : BusToVector
  Constant{2..6} (5 alike) : Constant  Value=0
  Step : Step  After=0  SampleTime=0
  "Disturbances " : Outport
  wires:
  Bus to Vector/1 -> "Disturbances "/1
  Bus Creator/1 -> Bus to Vector/1
  Constant6/1 -> Bus Creator/1  "Tau_bx-axis"
  Step/1 -> Bus Creator/2  "Tau_by-axis"
  Constant2/1 -> Bus Creator/3  "Tau_bz-axis"
  Constant3/1 -> Bus Creator/4  "Force_x-axis"
  Constant4/1 -> Bus Creator/5  "Force_y-axis"
  Constant5/1 -> Bus Creator/6  "Force_z-axis"

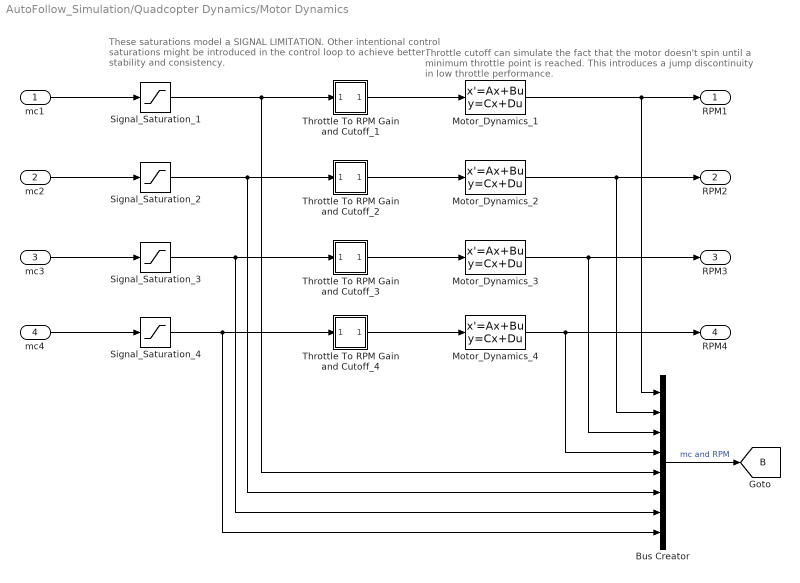
== system AutoFollow_Simulation/Quadcopter Dynamics/Motor Dynamics ==
  note: Throttle cutoff can simulate the fact that the motor doesn't
      | spin until a minimum throttle point is reached. This introduces
      | a jump discontinuity in low throttle performance.
  note: These saturations model a SIGNAL LIMITATION.
      | Other intentional control saturations might be introduced in the
      | control loop to achieve better stability and consistency.
  mc1 : Inport
  mc2 : Inport  Port=2
  mc3 : Inport  Port=3
  mc4 : Inport  Port=4
  Bus Creator : BusCreator  Inputs=8
  Motor_Dynamics_1 : StateSpace  A=-1/quadModel.T  C=1/quadModel.T  D=0  X0=IC.w1*quadModel.T
  Motor_Dynamics_2 : StateSpace  A=-1/quadModel.T  C=1/quadModel.T  D=0  X0=IC.w2*quadModel.T
  Motor_Dynamics_3 : StateSpace  A=-1/quadModel.T  C=1/quadModel.T  D=0  X0=IC.w3*quadModel.T
  Motor_Dynamics_4 : StateSpace  A=-1/quadModel.T  C=1/quadModel.T  D=0  X0=IC.w4*quadModel.T
  Signal_Saturation_{1..4} (4 alike) : Saturate  UpperLimit=100  LowerLimit=0
  Throttle To RPM Gain and Cutoff_1 : Subsystem
  Throttle To RPM Gain and Cutoff_2 : Subsystem
  Throttle To RPM Gain and Cutoff_3 : Subsystem
  Throttle To RPM Gain and Cutoff_4 : Subsystem
  RPM1 : Outport
  RPM2 : Outport  Port=2
  RPM3 : Outport  Port=3
  RPM4 : Outport  Port=4
  tag scope: B=global
  wires:
  mc1/1 -> Signal_Saturation_1/1
  mc4/1 -> Signal_Saturation_4/1
  mc2/1 -> Signal_Saturation_2/1
  mc3/1 -> Signal_Saturation_3/1
  Signal_Saturation_1/1 -> Bus Creator/5, Throttle To RPM Gain and Cutoff_1/1(In5)
  Signal_Saturation_2/1 -> Bus Creator/6, Throttle To RPM Gain and Cutoff_2/1(In5)
  Signal_Saturation_3/1 -> Bus Creator/7, Throttle To RPM Gain and Cutoff_3/1(In5)
  Signal_Saturation_4/1 -> Bus Creator/8, Throttle To RPM Gain and Cutoff_4/1(In5)
  Throttle To RPM Gain and Cutoff_1/1(Out5) -> Motor_Dynamics_1/1
  Throttle To RPM Gain and Cutoff_2/1(Out5) -> Motor_Dynamics_2/1
  Throttle To RPM Gain and Cutoff_3/1(Out5) -> Motor_Dynamics_3/1
  Throttle To RPM Gain and Cutoff_4/1(Out5) -> Motor_Dynamics_4/1
  Motor_Dynamics_1/1 -> Bus Creator/1, RPM1/1
  Motor_Dynamics_2/1 -> Bus Creator/2, RPM2/1
  Motor_Dynamics_3/1 -> Bus Creator/3, RPM3/1
  Motor_Dynamics_4/1 -> Bus Creator/4, RPM4/1
  Bus Creator/1 -> [B]  "mc and RPM"

== system AutoFollow_Simulation/Quadcopter Dynamics/Motor Dynamics/Throttle To RPM Gain and Cutoff_1 ==
  note: minThr should be a quad.mat value
  note: This gain should be a quad.mat value
  note: This constant should be a quad.mat value
  note: Output equals linearly scaled RPM
      | for given throttle input if throttle input >=Throttle Cuttoff (minThr)
      | else output is zero.
  In5 : Inport
  Constant : Constant  Value=quadModel.b
  Gain : Gain  Gain=quadModel.cr
  Minimum Throttle Cutoff : simulink/Logic and Bit Operations/Compare To Constant  relop=>=  const=quadModel.minThr  OutDataTypeStr=uint8
  Product : Product
  Sum1 : Sum  Inputs=++|
  Out5 : Outport
  wires:
  Minimum Throttle Cutoff/1 -> Product/2
  Product/1 -> Out5/1
  In5/1 -> Gain/1, Minimum Throttle Cutoff/1
  Gain/1 -> Sum1/2
  Sum1/1 -> Product/1
  Constant/1 -> Sum1/1

== system AutoFollow_Simulation/Quadcopter Dynamics/Motor Dynamics/Throttle To RPM Gain and Cutoff_2 ==
  note: minThr should be a quad.mat value
  note: This gain should be a quad.mat value
  note: This constant should be a quad.mat value
  note: Output equals linearly scaled RPM
      | for given throttle input if throttle input >=Throttle Cuttoff (minThr)
      | else output is zero.
  In5 : Inport
  Constant : Constant  Value=quadModel.b
  Gain : Gain  Gain=quadModel.cr
  Minimum Throttle Cutoff : simulink/Logic and Bit Operations/Compare To Constant  relop=>=  const=quadModel.minThr  OutDataTypeStr=uint8
  Product : Product
  Sum1 : Sum  Inputs=++|
  Out5 : Outport
  wires:
  Minimum Throttle Cutoff/1 -> Product/2
  Product/1 -> Out5/1
  In5/1 -> Gain/1, Minimum Throttle Cutoff/1
  Gain/1 -> Sum1/2
  Sum1/1 -> Product/1
  Constant/1 -> Sum1/1

== system AutoFollow_Simulation/Quadcopter Dynamics/Motor Dynamics/Throttle To RPM Gain and Cutoff_3 ==
  note: minThr should be a quad.mat value
  note: This gain should be a quad.mat value
  note: This constant should be a quad.mat value
  note: Output equals linearly scaled RPM
      | for given throttle input if throttle input >=Throttle Cuttoff (minThr)
      | else output is zero.
  In5 : Inport
  Constant : Constant  Value=quadModel.b
  Gain : Gain  Gain=quadModel.cr
  Minimum Throttle Cutoff : simulink/Logic and Bit Operations/Compare To Constant  relop=>=  const=quadModel.minThr  OutDataTypeStr=uint8
  Product : Product
  Sum1 : Sum  Inputs=++|
  Out5 : Outport
  wires:
  Minimum Throttle Cutoff/1 -> Product/2
  Product/1 -> Out5/1
  In5/1 -> Gain/1, Minimum Throttle Cutoff/1
  Gain/1 -> Sum1/2
  Sum1/1 -> Product/1
  Constant/1 -> Sum1/1

== system AutoFollow_Simulation/Quadcopter Dynamics/Motor Dynamics/Throttle To RPM Gain and Cutoff_4 ==
  note: minThr should be a quad.mat value
  note: This gain should be a quad.mat value
  note: This constant should be a quad.mat value
  note: Output equals linearly scaled RPM
      | for given throttle input if throttle input >=Throttle Cuttoff (minThr)
      | else output is zero.
  In5 : Inport
  Constant : Constant  Value=quadModel.b
  Gain : Gain  Gain=quadModel.cr
  Minimum Throttle Cutoff : simulink/Logic and Bit Operations/Compare To Constant  relop=>=  const=quadModel.minThr  OutDataTypeStr=uint8
  Product : Product
  Sum1 : Sum  Inputs=++|
  Out5 : Outport
  wires:
  Minimum Throttle Cutoff/1 -> Product/2
  Product/1 -> Out5/1
  In5/1 -> Gain/1, Minimum Throttle Cutoff/1
  Gain/1 -> Sum1/2
  Sum1/1 -> Product/1
  Constant/1 -> Sum1/1

== matlab function AutoFollow_Simulation/Camera/relativePosition ==
  data: xq input; yq input; zq input; thetaq input; psiq input; phiq input; hx input; hy input; hz input; r output; theta output; psi output; newMeas output
function [r, theta, psi, newMeas] = relativePosition(xq, yq, zq, thetaq, psiq, phiq, hx, hy, hz)
    persistent r_prev 
    persistent theta_prev
    persistent psi_prev
     
    %check if there's an obstacle between human and quadcopter.
    Xmax = 25; Ymax = 25;
    map = load('./Lidar/ObstacleMap/obstaclemap.mat'); % obstacle map
%     map = load('./Lidar/ObstacleMap/clearmap.mat');   % Clear map
    map = map.map;
    [R, C] = size(map);
    [Iq, Jq] = XYtoIJ(xq*3.28, yq*3.28, Xmax, Ymax, R, C);
    [Ih, Jh] = XYtoIJ(hx, hy, Xmax, Ymax, R, C);
    Pxel = laserRange([Iq Jq], [Ih Jh], map);
    [xCheck, yCheck] = IJtoXY(Pxel(1), Pxel(2), Xmax, Ymax, R, C);
    distCheck = sqrt((xq*3.28 - xCheck)^2 + (yq*3.28 - yCheck)^2);
    distHuman = sqrt((xq*3.28 - hx)^2 + (yq*3.28 - hy)^2);
    
    %if the obstacle is closer than the human use previous values
    if isempty(r_prev) || (distHuman < distCheck)
        %% first find relative vector from quadcopter to human
        p_not_rot = [xq*3.28 - hx; yq*3.28 - hy; zq*3.28 - hz];

        %% rotate person vector into quadcopter coordinates
        R = [cos(psiq)*cos(thetaq) cos(psiq)*sin(thetaq)*sin(phiq)-sin(psiq)*cos(phiq) cos(psiq)*sin(thetaq)*cos(phiq)+sin(psiq)*sin(phiq);
             sin(psiq)*cos(thetaq) sin(psiq)*sin(thetaq)*sin(phiq)+cos(psiq)*cos(phiq) sin(psiq)*sin(thetaq)*cos(phiq)-cos(psiq)*sin(phiq);
             -sin(thetaq)          cos(thetaq)*sin(phiq)                               cos(thetaq)*cos(phiq)];

        p = (R^-1)*p_not_rot;

        %% transform p into sphereichumanMovementTestal coordinates
        % x = r * sin(p) * cos(t) 
        % y = r * sin(p) * sin(t) 
        % z = r * cos(p) 
        % If you already have x,y,z and want to switch it back, this is the conversion: 
        % r = sqrt(x*x + y*y + z*z) 
        % theta = arctan(y/x)
        % psi = arccos(z/r)
        r = sqrt(sum(p.^2));
        theta = atan2(p(2),p(1));
        psi = acos(p(3)/r);  %Should be asin(p/r) for pitch angle (theta not psi)
        newMeas = 1;
        
        r_prev = r;
        theta_prev = theta;
        psi_prev = psi;

        %% debugging!!
    %     %same process as in plotting (to reverse the 'camera coordinates')
    %     cam_x = r.*sin(psi).*cos(theta);
    %     cam_y = r.*sin(psi).*sin(theta);
    %     cam_z = r.*cos(psi);
    %     Rback = [cos(psiq)*cos(thetaq) cos(psiq)*sin(thetaq)*sin(phiq)-sin(psiq)*cos(phiq) cos(psiq)*sin(thetaq)*cos(phiq)+sin(psiq)*sin(phiq);
    %               sin(psiq)*cos(thetaq) sin(psiq)*sin(thetaq)*sin(phiq)+cos(psiq)*cos(phiq) sin(psiq)*sin(thetaq)*cos(phiq)-cos(psiq)*sin(phiq);
    %               -sin(thetaq)         cos(thetaq)*sin(phiq)                            cos(thetaq)*cos(phiq)];
    %     cam = [cam_x; cam_y; cam_z];
    %     human_cam = Rback*cam;
    %     if (hx > 1)
    %     lol = 1;
    %     end
    else
        %use previous
        r = r_prev;
        theta = theta_prev;
        psi = psi_prev;
        newMeas = 0;
    end
end

== matlab function AutoFollow_Simulation/PathCommandMatt /MATLAB Function ==
  data: Chi input; X output size=1; Y output; Z output; Psi output; xH input; yH input; zH input; R_L input; theta_L input; t input
function [X,Y,Z,Psi]   = PathPlannerFunBlock(Chi,xH,yH,zH,R_L,theta_L,t)
%% Questions:
% What is theta_c and Psi_c in camera block. They seem backwards?
% I need a yaw angle of camera wrt vehicle 1 frame or vehhicle frame?
% Quadcopter in meters, graphing and human are in feet.
% States [x, y, z, psi,time] of robot
% Camera data = [R_c, psi_c]


R        = 4;      % ft, desired radius of path
% %% Undo spherical coordinates for human position rel. to copter
% % human vector in body fixed frame is in spherical coordinates, undo for
% % using these equations
%     % x = r * sin(p) * cos(t) 
%     % y = r * sin(p) * sin(t) 
%     % z = r * cos(p) 
% p_quad = zeros(3,1);
% p_quad(1) = (R_c)*sin(psi_c)*cos(theta_c);
% p_quad(2) = (R_c)*sin(psi_c)*sin(theta_c); 
% p_quad(3) =  R_c*cos(psi_c);
% 
% % rotate human position into global points
% Rot = [cos(psiq)*cos(thetaq) cos(psiq)*sin(thetaq)*sin(phiq)-sin(psiq)*cos(phiq) cos(psiq)*sin(thetaq)*cos(phiq)+sin(psiq)*sin(phiq);
%        sin(psiq)*cos(thetaq) sin(psiq)*sin(thetaq)*sin(phiq)+cos(psiq)*cos(phiq) sin(psiq)*sin(thetaq)*cos(phiq)-cos(psiq)*sin(phiq);
%        -sin(thetaq)          cos(thetaq)*sin(phiq)                               cos(thetaq)*cos(phiq)];
%     
% p_global = Rot*p_quad;
% 
% % Human pos. rel. to quadcopter
xH = -xH;
yH = -yH;
zH = -zH;

% Goal position relative to quad vehicle frame
% ( x horz, y vertical) /3.28 convert feet to meters for quad sim
x_g = xH/3.28 - R(1)/3.28084*cos(Chi);
y_g = yH/3.28 - R(1)/3.28084*sin(Chi);

% Attractive Force
eps = 1;
C_A = 0.5; % attractive constant
d_a = sqrt(x_g^2 + y_g^2); % normalizing distance to goal position
F_Ax = C_A * x_g/(d_a + eps); 
F_Ay = C_A * y_g/(d_a + eps);


% Repulsive Force and Lidar data
R_L = R_L / 3.28; % convert ft to meters
% Find maximumn laser reading (if reading returns max, no obstacle)
maxR_L = max(R_L);
C_R = 0.3;
rho = 2;
% obstalce location
count = 1;
F_Rx = 0;
F_Ry = 0;
for i = 1:length(R_L)
    if R_L(i) < maxR_L % obstaacle here
        x_o = R_L(i)*cos(theta_L(i));
        y_o = R_L(i)*sin(theta_L(i));
        d_o = sqrt(x_o^2 + y_o^2);
        F_Rx = F_Rx + C_R * x_o/(d_o)^rho;
        F_Ry = F_Ry + C_R * y_o/(d_o)^rho;
        count = count + 1;
    end
end
% use average repulsive force from all obstacles detected
F_Rx = (F_Rx)/count;
F_Ry = (F_Ry)/count;

% combine forces to output new goal position
X = F_Ax + F_Rx;
Y = F_Ay + F_Ry;
if t > 25
    cat = 8;
end


% height
Z = 10/3.28; % feet
Psi = pi/2;%Chi; % yaw angle same as chi


end

== matlab function AutoFollow_Simulation/Lidar/MATLAB Function ==
  data: xq input; r output; yq input; theta output; t input
function [r,theta] = fcn(xq, yq, t)
    persistent prev_t;
    persistent prev_r;
    persistent prev_theta;

    if isempty(prev_t)
        prev_t = 0;
    end

    %will initialize, and only run lidar update every X seconds
    lidarUpdateTime = 0.1;
    if (isempty(prev_r) || (t - prev_t) > lidarUpdateTime)
        % min and max of world coordinates (sees obtacle at edge)
        Xmax = 25; Ymax = 25;
        map = load('./Lidar/ObstacleMap/obstaclemap.mat'); % obstacle map
%         map = load('./Lidar/ObstacleMap/clearmap.mat');   % Clear map
        map = map.map;
        % span of scanner and step size
        angleSpan = 2*pi; angleStep = 2*pi/360;
        %(m) max range of lidar scanner 
        rangeMax=50; 
        %current laser pose (coordinate frame) wrt world
        % Laser located in vehcile frame of quadcopter
        Tl=se2([xq*3.28 yq*3.28 0]); 

        % p = laserScanner(angleSpan, angleStep, rangeMax, Tl, map, Xmin, Ymin, Xmax, Ymax)
        % return (theta,r) of scan
        p = laserScanner(angleSpan, angleStep, rangeMax, Tl, map, Xmax, Ymax); %p contains angle and range readings

        % figure(2);
        % plot(p(:,1)*180/pi, p(:,2)); % plot angle and range - it is displayed in ccw, from -angleSpan/2 to +angleSpan/2

        r = p(:,2); theta = p(:,1) + deg2rad(180);
        prev_r = r;
        prev_theta = theta;
        prev_t = t;
    else
        r = prev_r;
        theta = prev_theta;
    end
end
